simulink model "driver_led_indication_RL"  (R2024a)
settings: Solver=FixedStepAuto  StartTime=0.0  StopTime=10  MaxStep=1e-3  RelTol=1e-3  EnableMultiTasking=on
libraries: arduinolib x5, simulink x1
settings Model: ExtModeTrigDuration=2  Creator=DELL  LastModifiedBy=DELL
settings SolverCC: AutoInsertRateTranBlk=on
settings OptimizationCC: EnhancedBackFolding=on  PassReuseOutputArgsAs=Individual arguments  ZeroExternalMemoryAtStartup=off  ZeroInternalMemoryAtStartup=off  MaxStackSize=64  OptimizeBlockOrder=speed  DifferentSizesBufferReuse=on  OptimizationCustomize=off  EfficientTunableParamExpr=on
settings DebuggingCC: ParameterTunabilityLossMsg=error
settings HardwareCC: ProdBitPerInt=16  ProdBitPerPointer=16  ProdBitPerSizeT=16  ProdBitPerPtrDiffT=16  ProdLargestAtomicFloat=None  ProdWordSize=8  ProdHWDeviceType=Atmel->AVR
settings SFSimCC: MATLABDynamicMemAlloc=off
settings RTWCC: Description=Embedded Coder  SystemTargetFile=ert.tlc  HardwareBoard=Arduino Uno  TemplateMakefile=ert_default_tmf  Toolchain=Arduino AVR  BuildConfiguration=Faster Runs
settings CodeAppCC: ForceParamTrailComments=on  IgnoreCustomStorageClasses=off  OperatorAnnotations=on  SimulinkDataObjDesc=on  SFDataObjDesc=on  InsertBlockDesc=on
settings ERTTargetCC: SupportContinuousTime=on  SupportVariableSizeSignals=on  ExtModeTransport=3  ExtModeStaticAlloc=on  ExtModeAutomaticAllocSize=off  ExtModeStaticAllocSize=250  ExtModeMexFile=ext_xcp  ExtModeIntrfLevel=Level2 - Open

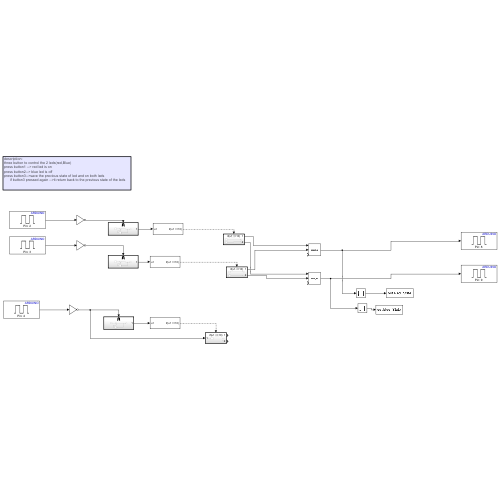
[thumbnail: Simulink's stored preview of the top-level diagram]
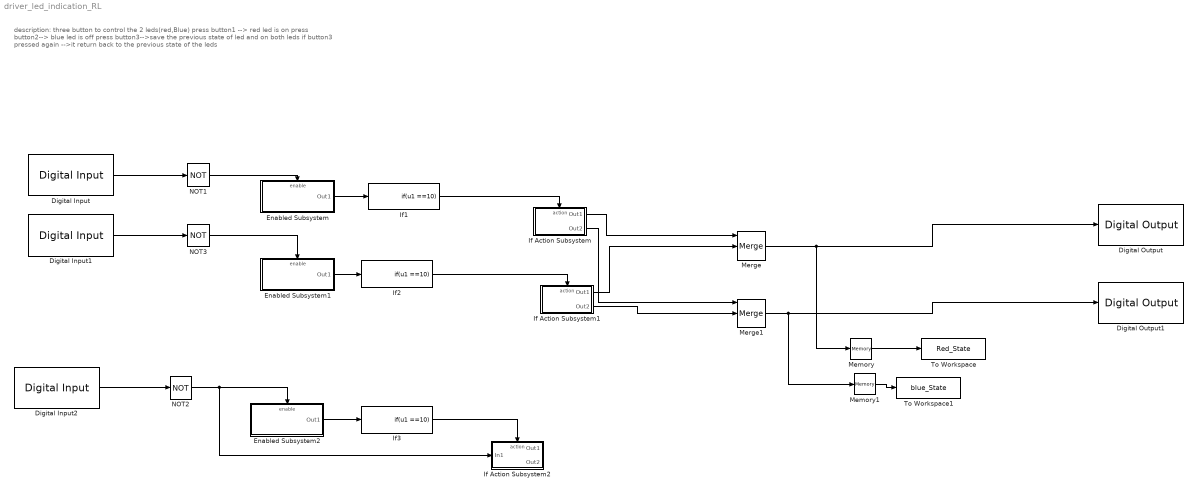
== system driver_led_indication_RL ==
  note: description:
      | three button to control the 2 leds(red,Blue)
      | press button1 --> red led is on
      | press button2--> blue led is off
      | press button3-->save the previous state of led and on both leds
      | 	if button3 pressed again -->it return back to the previous state of the leds
  Digital Input : arduinolib/Digital Input  pinNumber=2  mode=Input Pullup  Direction=input  SampleTime=0.1  blockPlatform=arduino
  Digital Input1 : arduinolib/Digital Input  pinNumber=3  mode=Input Pullup  Direction=input  SampleTime=0.1  blockPlatform=arduino
  Digital Input2 : arduinolib/Digital Input  pinNumber=4  mode=Input Pullup  Direction=input  SampleTime=0.1  blockPlatform=arduino
  Digital Output : arduinolib/Digital Output  pinNumber=8  Direction=output  blockPlatform=arduino
  Digital Output1 : arduinolib/Digital Output  pinNumber=9  Direction=output  blockPlatform=arduino
  Enabled Subsystem : Subsystem  TreatAsAtomicUnit=on
  Enabled Subsystem1 : Subsystem  TreatAsAtomicUnit=on
  Enabled Subsystem2 : Subsystem  TreatAsAtomicUnit=on
  If Action Subsystem : Subsystem  TreatAsAtomicUnit=on
  If Action Subsystem1 : Subsystem  TreatAsAtomicUnit=on
  If Action Subsystem2 : Subsystem  TreatAsAtomicUnit=on
  If1 : If  IfExpression=u1 ==10  ShowElse=off
  If2 : If  IfExpression=u1 ==10  ShowElse=off
  If3 : If  IfExpression=u1 ==10  ShowElse=off
  Memory : Memory
  Memory1 : Memory
  Merge : Merge  Inputs=3
  Merge1 : Merge  Inputs=3
  NOT1 : Logic  Operator=NOT  IconShape=distinctive  AllPortsSameDT=off  OutDataTypeStr=boolean
  NOT2 : Logic  Operator=NOT  IconShape=distinctive  AllPortsSameDT=off  OutDataTypeStr=boolean
  NOT3 : Logic  Operator=NOT  IconShape=distinctive  AllPortsSameDT=off  OutDataTypeStr=boolean
  To Workspace : ToWorkspace  VariableName=Red_State  SaveFormat=Timeseries  SampleTime=-1
  To Workspace1 : ToWorkspace  VariableName=blue_State  SaveFormat=Timeseries  SampleTime=-1
  wires:
  Digital Input2/1 -> NOT2/1
  Digital Input/1 -> NOT1/1
  Digital Input1/1 -> NOT3/1
  NOT1/1 -> Enabled Subsystem/Enable
  Enabled Subsystem/1(Out1) -> If1/1
  Enabled Subsystem1/1(Out1) -> If2/1
  NOT3/1 -> Enabled Subsystem1/Enable
  If1/1 -> If Action Subsystem/Action
  If2/1 -> If Action Subsystem1/Action
  Enabled Subsystem2/1(Out1) -> If3/1
  If3/1 -> If Action Subsystem2/Action
  NOT2/1 -> If Action Subsystem2/1(In1), Enabled Subsystem2/Enable
  If Action Subsystem/1(Out1) -> Merge/1
  If Action Subsystem/2(Out2) -> Merge1/1
  If Action Subsystem1/1(Out1) -> Merge/2
  If Action Subsystem1/2(Out2) -> Merge1/2
  Merge/1 -> Memory/1, Digital Output/1
  Merge1/1 -> Memory1/1, Digital Output1/1
  Memory/1 -> To Workspace/1
  Memory1/1 -> To Workspace1/1

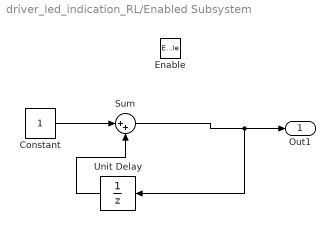
== system driver_led_indication_RL/Enabled Subsystem ==
  Enable : EnablePort  StatesWhenEnabling=reset
  Constant : Constant
  Sum : Sum  Inputs=|++
  Unit Delay : UnitDelay  SampleTime=-1  HasFrameUpgradeWarning=on
  Out1 : Outport
  wires:
  Constant/1 -> Sum/1
  Unit Delay/1 -> Sum/2
  Sum/1 -> Unit Delay/1, Out1/1

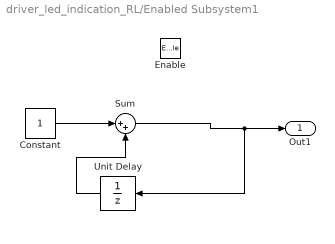
== system driver_led_indication_RL/Enabled Subsystem1 ==
  Enable : EnablePort  StatesWhenEnabling=reset
  Constant : Constant
  Sum : Sum  Inputs=|++
  Unit Delay : UnitDelay  SampleTime=-1  HasFrameUpgradeWarning=on
  Out1 : Outport
  wires:
  Sum/1 -> Out1/1, Unit Delay/1
  Unit Delay/1 -> Sum/2
  Constant/1 -> Sum/1

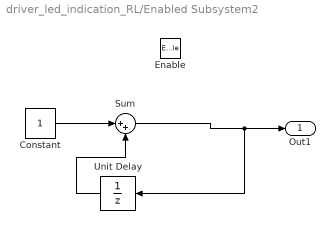
== system driver_led_indication_RL/Enabled Subsystem2 ==
  Enable : EnablePort  StatesWhenEnabling=reset
  Constant : Constant
  Sum : Sum  Inputs=|++
  Unit Delay : UnitDelay  SampleTime=-1  HasFrameUpgradeWarning=on
  Out1 : Outport
  wires:
  Sum/1 -> Out1/1, Unit Delay/1
  Unit Delay/1 -> Sum/2
  Constant/1 -> Sum/1

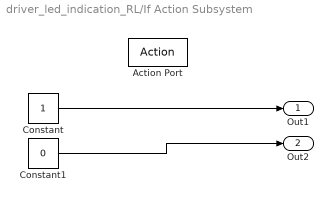
== system driver_led_indication_RL/If Action Subsystem ==
  Action Port : ActionPort  ActionPortLabel=if(u1 ==10)
  Constant : Constant
  Constant1 : Constant  Value=0
  Out1 : Outport
  Out2 : Outport  Port=2
  wires:
  Constant/1 -> Out1/1
  Constant1/1 -> Out2/1

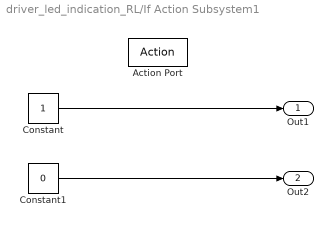
== system driver_led_indication_RL/If Action Subsystem1 ==
  Action Port : ActionPort  ActionPortLabel=if(u1 ==10)
  Constant : Constant
  Constant1 : Constant  Value=0
  Out1 : Outport
  Out2 : Outport  Port=2
  wires:
  Constant/1 -> Out1/1
  Constant1/1 -> Out2/1

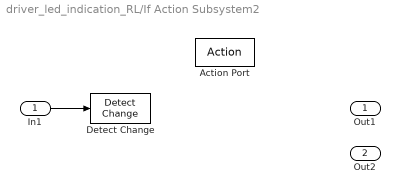
== system driver_led_indication_RL/If Action Subsystem2 ==
  In1 : Inport
  Action Port : ActionPort  ActionPortLabel=if(u1 ==10)
  Detect Change : simulink/Logic and Bit Operations/Detect Change  vinit=0  OutDataTypeStr=boolean
  Out1 : Outport
  Out2 : Outport  Port=2
  wires:
  In1/1 -> Detect Change/1
